simulink model "ejemplo1"  (R2025b)
settings: Solver=VariableStepAuto  StartTime=0.0  StopTime=10.0  RelTol=1e-3

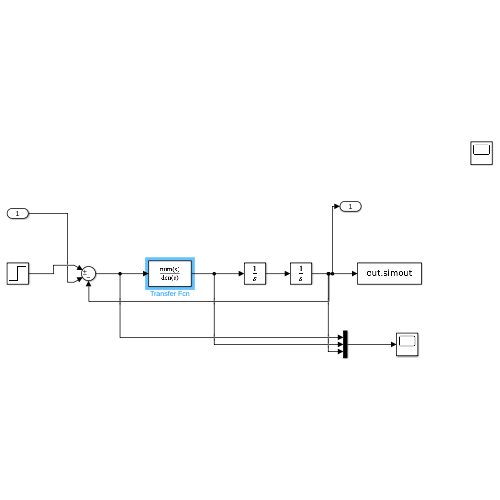
[thumbnail: Simulink's stored preview of the top-level diagram]
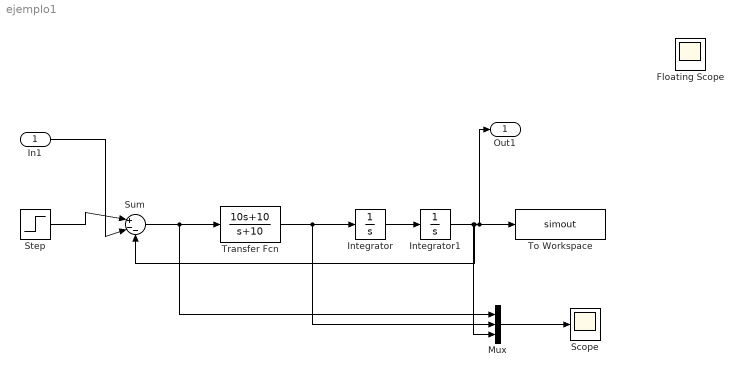
== system ejemplo1 ==
  In1 : Inport
  Floating Scope : Scope
      settings: IsFloating=on  Floating=on  ActiveDisplayYMinimum=-12.398784844335655  ActiveDisplayYMaximum=10.753715155664349
  Integrator : Integrator
  Integrator1 : Integrator
  Mux : Mux  Inputs=3
  Scope : Scope
  Step : Step  SampleTime=0
  Sum : Sum  Inputs=|+--
  To Workspace : ToWorkspace  VariableName=simout  SaveFormat=Timeseries  SampleTime=-1
  Transfer Fcn : TransferFcn  Numerator=[10 10]  Denominator=[1 10]
  Out1 : Outport
  wires:
  Step/1 -> Sum/1
  In1/1 -> Sum/2
  Sum/1 -> Mux/1, Transfer Fcn/1
  Transfer Fcn/1 -> Mux/2, Integrator/1
  Integrator/1 -> Integrator1/1
  Mux/1 -> Scope/1
  Integrator1/1 -> To Workspace/1, Out1/1, Sum/3, Mux/3
